simulink model "SplineGeneratorTest"  (R2016b)
settings: Solver=VariableStepAuto  StartTime=0.0  StopTime=10.0  RelTol=1e-3
settings Model: Creator=march  LastModifiedBy=Taeke

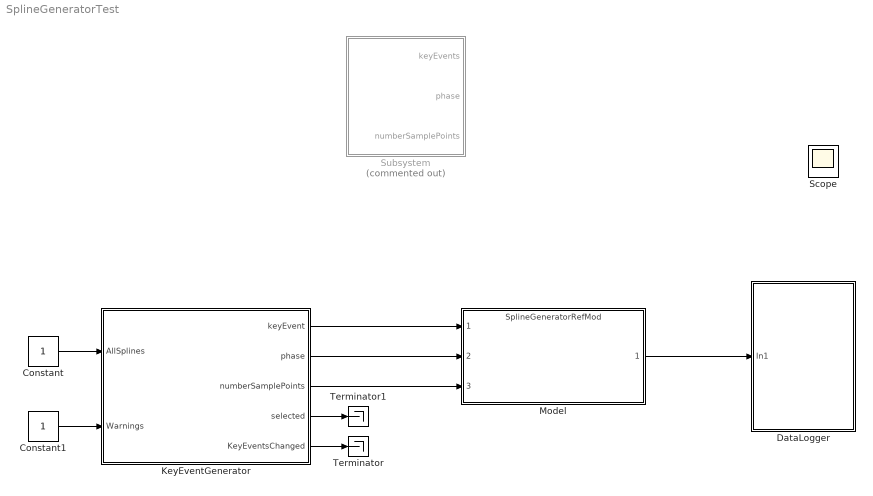
== system SplineGeneratorTest ==
  Constant : Constant
  Constant1 : Constant
  DataLogger : Subsystem  AncestorBlock=GaitGenerationLibrary/DataLogger
  KeyEventGenerator : Subsystem  AncestorBlock=GaitGenerationLibrary/KeyEventGenerator
  Model : ModelReference  ModelNameDialog=SplineGeneratorRefMod.slx  SimulationMode=Normal  ModelReferenceVersion=1.18
  Scope : Scope
  Subsystem : Subsystem  Commented=on
  Terminator : Terminator
  Terminator1 : Terminator
  wires:
  KeyEventGenerator/1(keyEvent) -> Model/1
  KeyEventGenerator/2(phase) -> Model/2
  KeyEventGenerator/3(numberSamplePoints) -> Model/3
  KeyEventGenerator/5(KeyEventsChanged) -> Terminator/1
  Constant/1 -> KeyEventGenerator/1(AllSplines)
  Constant1/1 -> KeyEventGenerator/2(Warnings)
  Model/1 -> DataLogger/1(In1)
  KeyEventGenerator/4(selected) -> Terminator1/1

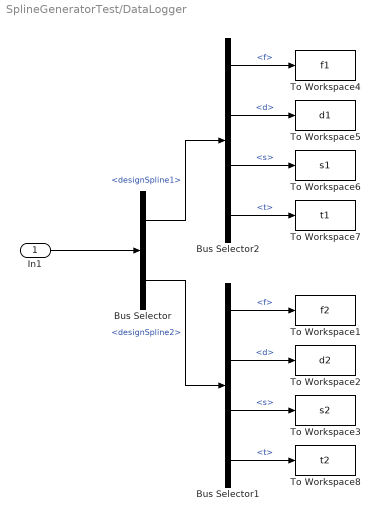
== system SplineGeneratorTest/DataLogger ==
  In1 : Inport
  Bus Selector : BusSelector  OutputSignals=designSpline1,designSpline2
  Bus Selector1 : BusSelector  OutputSignals=f,d,s,t
  Bus Selector2 : BusSelector  OutputSignals=f,d,s,t
  To Workspace1 : ToWorkspace  VariableName=f2  SaveFormat=Timeseries  SampleTime=-1
  To Workspace2 : ToWorkspace  VariableName=d2  SaveFormat=Timeseries  SampleTime=-1
  To Workspace3 : ToWorkspace  VariableName=s2  SaveFormat=Timeseries  SampleTime=-1
  To Workspace4 : ToWorkspace  VariableName=f1  SaveFormat=Timeseries  SampleTime=-1
  To Workspace5 : ToWorkspace  VariableName=d1  SaveFormat=Timeseries  SampleTime=-1
  To Workspace6 : ToWorkspace  VariableName=s1  SaveFormat=Timeseries  SampleTime=-1
  To Workspace7 : ToWorkspace  VariableName=t1  SaveFormat=Timeseries  SampleTime=-1
  To Workspace8 : ToWorkspace  VariableName=t2  SaveFormat=Timeseries  SampleTime=-1
  wires:
  In1/1 -> Bus Selector/1
  Bus Selector/2 -> Bus Selector1/1  "<designSpline2>"
  Bus Selector/1 -> Bus Selector2/1  "<designSpline1>"
  Bus Selector2/1 -> To Workspace4/1  "<f>"
  Bus Selector2/2 -> To Workspace5/1  "<d>"
  Bus Selector2/3 -> To Workspace6/1  "<s>"
  Bus Selector2/4 -> To Workspace7/1  "<t>"
  Bus Selector1/1 -> To Workspace1/1  "<f>"
  Bus Selector1/2 -> To Workspace2/1  "<d>"
  Bus Selector1/3 -> To Workspace3/1  "<s>"
  Bus Selector1/4 -> To Workspace8/1  "<t>"

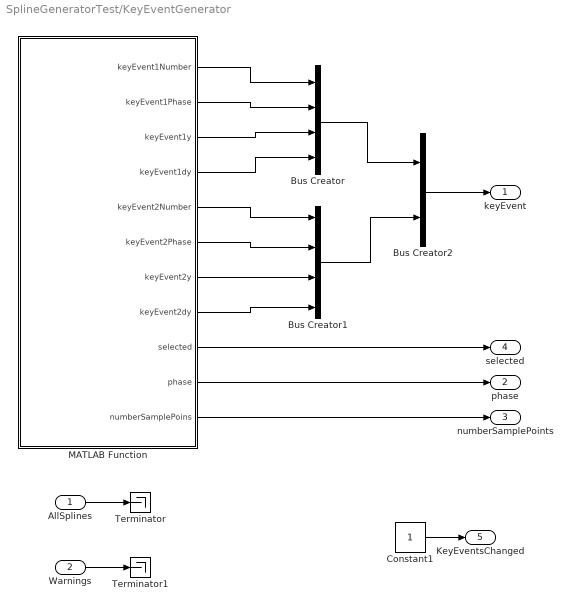
== system SplineGeneratorTest/KeyEventGenerator ==
  AllSplines : Inport
  Warnings : Inport  Port=2
  Bus Creator : BusCreator  Inputs=4  OutDataTypeStr=Bus: keyEvent1
  Bus Creator1 : BusCreator  Inputs=4  OutDataTypeStr=Bus: keyEvent2
  Bus Creator2 : BusCreator  Inputs=2
  Constant1 : Constant
  MATLAB Function : MATLAB Function  TreatAsAtomicUnit=on
  Terminator : Terminator
  Terminator1 : Terminator
  keyEvent : Outport
  phase : Outport  Port=2
  numberSamplePoints : Outport  Port=3
  selected : Outport  Port=4
  KeyEventsChanged : Outport  Port=5
  wires:
  MATLAB Function/4(keyEvent1dy) -> Bus Creator/4
  MATLAB Function/3(keyEvent1y) -> Bus Creator/3
  MATLAB Function/2(keyEvent1Phase) -> Bus Creator/2
  MATLAB Function/1(keyEvent1Number) -> Bus Creator/1
  MATLAB Function/10(phase) -> phase/1
  MATLAB Function/11(numberSamplePoins) -> numberSamplePoints/1
  Warnings/1 -> Terminator1/1
  AllSplines/1 -> Terminator/1
  Constant1/1 -> KeyEventsChanged/1
  MATLAB Function/8(keyEvent2dy) -> Bus Creator1/4
  MATLAB Function/7(keyEvent2y) -> Bus Creator1/3
  MATLAB Function/6(keyEvent2Phase) -> Bus Creator1/2
  MATLAB Function/5(keyEvent2Number) -> Bus Creator1/1
  Bus Creator1/1 -> Bus Creator2/2
  Bus Creator2/1 -> keyEvent/1
  MATLAB Function/9(selected) -> selected/1
  Bus Creator/1 -> Bus Creator2/1

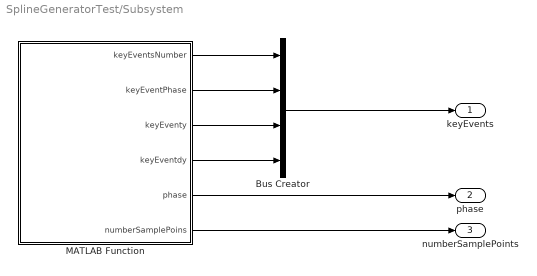
== system SplineGeneratorTest/Subsystem ==
  Bus Creator : BusCreator  Inputs=4
  MATLAB Function : MATLAB Function  TreatAsAtomicUnit=on
  keyEvents : Outport
  phase : Outport  Port=2
  numberSamplePoints : Outport  Port=3
  wires:
  MATLAB Function/6(numberSamplePoins) -> numberSamplePoints/1
  MATLAB Function/5(phase) -> phase/1
  Bus Creator/1 -> keyEvents/1
  MATLAB Function/1(keyEventsNumber) -> Bus Creator/1
  MATLAB Function/2(keyEventPhase) -> Bus Creator/2
  MATLAB Function/3(keyEventy) -> Bus Creator/3
  MATLAB Function/4(keyEventdy) -> Bus Creator/4

== matlab function SplineGeneratorTest/Subsystem/MATLAB Function ==
  data: keyEventsNumber output; keyEventPhase output; keyEventy output; keyEventdy output; phase output; numberSamplePoins output
function [keyEventsNumber, keyEventPhase,keyEventy,keyEventdy, phase, numberSamplePoins] = fcn()

keyEventPhase = [0, 20, 40, 60, 80, 100];
keyEventy = [0, 40, 30, -10, -10, 0];
keyEventdy = [0,-1,-1,0,1,0];

phase = (0:0.1:100)';

numberSamplePoins = 100;

keyEventsNumber = length(KeyEventPhase);
end

== matlab function SplineGeneratorTest/KeyEventGenerator/MATLAB Function ==
  data: keyEvent1Number output; keyEvent1Phase output; keyEvent1y output; keyEvent1dy output; keyEvent2Number output; keyEvent2Phase output; keyEvent2y output; keyEvent2dy output; selected output; phase output; numberSamplePoins output
function [keyEvent1Number, keyEvent1Phase,keyEvent1y,keyEvent1dy, ...
    keyEvent2Number, keyEvent2Phase,keyEvent2y,keyEvent2dy,...
    selected, phase, numberSamplePoins] = fcn()

keyEvent1Phase = [0, 20, 40, 60, 80, 100];
keyEvent1y = [0, 40, 30, -10, -10, 0];
keyEvent1dy = [0,-1,-1,0,1,0];
keyEvent1Number = length(keyEvent1Phase);

keyEvent2Phase = [0, 20, 40, 60, 80, 100];
keyEvent2y = [-20, 30, 90, 100, 20, 0];
keyEvent2dy = [0,1,1,-1,-1,0];
keyEvent2Number = length(keyEvent2Phase);

selected = [1, 1, 0, 0];

phase = (0:0.1:100)';

numberSamplePoins = 100;


end
